simulink model "lab4_3_"  (R2023a)
settings: Solver=VariableStepAuto  StartTime=0.0  StopTime=50  RelTol=1e-3
values from neighbouring files (symbols this model uses):
  kd = 0.48315    [lab4_3.m]
  ki = 1.8463    [lab4_3.m]
  kp = 1.1776    [lab4_3.m]
libraries: checkpacklib x2, slpidlib x1
settings Model: Creator=diontep  LastModifiedBy=diontep

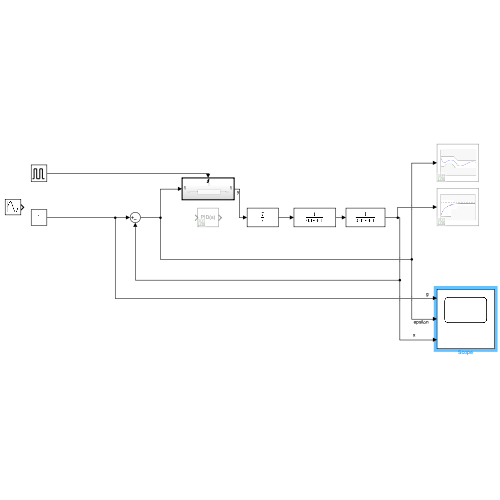
[thumbnail: Simulink's stored preview of the top-level diagram]
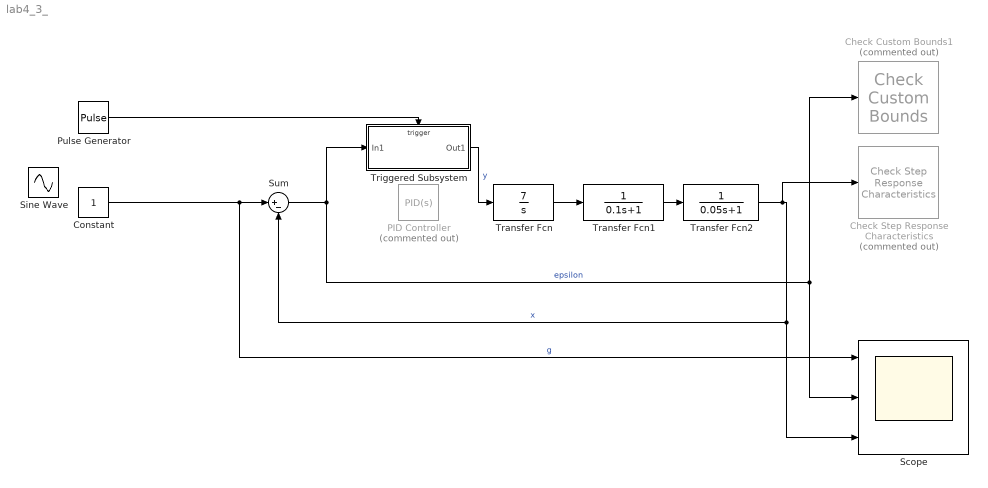
== system lab4_3_ ==
  Check Custom Bounds1 : checkpacklib/Check Custom Bounds  Commented=on  InstantiateOnLoad=on  enabled=on  stopWhenAssertionFail=off  export=off  ViewDlgPos=[]  OpenViewOnLoad=off  LaunchViewOnOpen=off  TimeUnits=seconds  EnableUpperBound=on  UpperBoundTimes=[0 5; 5 50]  UpperBoundAmplitudes=[10 10; 1 1];  EnableLowerBound=on  LowerBoundTimes=[0 5; 5 50]  LowerBoundAmplitudes=[-10 -10; -1 -1];
      settings: LibrarySourceBlock=sdolib/Signal Constraints/Check Custom Bounds
  Check Step Response Characteristics : checkpacklib/Check Step Response  Characteristics  Commented=on  InstantiateOnLoad=on  enabled=on  stopWhenAssertionFail=off  export=off  ViewDlgPos=[]  OpenViewOnLoad=off  LaunchViewOnOpen=off  TimeUnits=seconds  EnableStepResponseBound=on  InitialValue=0  FinalValue=1  StepTime=0  RiseTime=5  PercentRise=80  SettlingTime=7  PercentSettling=1  PercentOvershoot=10  PercentUndershoot=1
      settings: LibrarySourceBlock=|
      | sdolib/Signal Constraints/Check Step Response
      | Characteristics
  Constant : Constant
  PID Controller : slpidlib/PID Controller  Commented=on  Controller=PID  Form=Parallel  TimeDomain=Continuous-time  UseExternalTs=off  SampleTime=-1  IntegratorMethod=Forward Euler  FilterMethod=Forward Euler  ControllerParametersSource=internal  P=kp  I=ki  UseKiTs=off  D=kd  N=100  UseFilter=on  TunerSelectOption=Transfer Function Based (PID Tuner App)  InitialConditionSource=internal  InitialConditionForIntegrator=0  InitialConditionForFilter=0  DifferentiatorICPrevScaledInput=0  ExternalReset=none  TrackingMode=off  Kt=1  LimitOutput=off  SatLimitsSource=internal  UpperSaturationLimit=inf  LowerSaturationLimit=-inf  LinearizeAsGain=on  AntiWindupMode=none  Kb=1  LimitIntegrator=off  UpperIntegratorSaturationLimit=inf  LowerIntegratorSaturationLimit=-inf  POutMin=[]  POutMax=[]  IOutMin=[]  IOutMax=[]  DOutMin=[]  DOutMax=[]  NOutMin=[]  NOutMax=[]  SumOutMin=[]  SumOutMax=[]  SaturationOutMin=[]  SaturationOutMax=[]  PParamMin=[]  PParamMax=[]  IParamMin=[]  IParamMax=[]  DParamMin=[]  DParamMax=[]  NParamMin=[]  NParamMax=[]  KbParamMin=[]  KbParamMax=[]  KtParamMin=[]  KtParamMax=[]  KbOutMin=[]  KbOutMax=[]  KtOutMin=[]  KtOutMax=[]  IntegratorOutMin=[]  IntegratorOutMax=[]  FilterOutMin=[]  FilterOutMax=[]  SumI1OutMin=[]  SumI1OutMax=[]  SumI2OutMin=[]  SumI2OutMax=[]  SumI3OutMin=[]  SumI3OutMax=[]  SumI4OutMin=[]  SumI4OutMax=[]  SumDOutMin=[]  SumDOutMax=[]  DifferentiatorOutMin=[]  DifferentiatorOutMax=[]  FilterDiffOutCoefMin=[]  FilterDiffOutCoefMax=[]  ReciprocalOutMin=[]  ReciprocalOutMax=[]  SumDenOutMin=[]  SumDenOutMax=[]  SumNumOutMin=[]  SumNumOutMax=[]  DivideOutMin=[]  DivideOutMax=[]  UdiffTsProdOutMin=[]  UdiffTsProdOutMax=[]  NTsProdOutMin=[]  NTsProdOutMax=[]  UintegralTsProdOutMin=[]  UintegralTsProdOutMax=[]  UngainTsProdOutMin=[]  UngainTsProdOutMax=[]  ClampingZeroOutDataTypeStr=Inherit: Inherit via back propagation  ClampingZeroOutMin=[]  ClampingZeroOutMax=[]  FilterDenConstantOutDataTypeStr=Inherit: Inherit via back propagation  FilterDenConstantOutMin=[]  FilterDenConstantOutMax=[]  PCopyOutDataTypeStr=Inherit: Inherit via back propagation  PCopyOutMin=[]  PCopyOutMax=[]  NCopyOutDataTypeStr=Inherit: Inherit via back propagation  NCopyOutMin=[]  NCopyOutMax=[]  IntegratorContinuousStateAttributes=''  IntegratorStateMustResolveToSignalObject=off  IntegratorRTWStateStorageClass=Auto  FilterContinuousStateAttributes=''  FilterStateMustResolveToSignalObject=off  FilterRTWStateStorageClass=Auto  ParallelPVariant=InternalParameters  IdealPVariant=Disabled  IVariant=InternalParameters  DVariant=InternalParameters  IntegratorVariant=Continuous  SatVariant=Disabled  AWVariant=Passthrough  PCopyVariant=Disabled  TRVariant=Disabled  FdbkBlocksVariant=Forward  IdealPFdbkVariant=Disabled  SatFdbkVariant=Disabled  DerivativeFilterVariant=ContFilter  NVariant=InternalParameters  NCopyVariant=Disabled  FilterICVariant=InternalICsFilter  IntegratorICVariant=InternalICs  ExternalResetVariant=Disabled  TRSumVariant=Passthrough  SumFdbkVariant=Disabled  SumVariant=Sum_PID  TsampFilterVariant=InternalTs  TsampNgainVariant=Passthrough  TsampIntegralVariant=Disabled_SignalSpec  ExternalSaturationOutDataTypeStr=Inherit: Same as second input
  Pulse Generator : DiscretePulseGenerator  PulseType=Time based  Period=0.01  PulseWidth=50
  Scope : Scope  NumInputPorts=3
  Sine Wave : Sin  Amplitude=50  Frequency=0.5  SampleTime=0
  Sum : Sum  Inputs=|+-
  Transfer Fcn : TransferFcn  Numerator=[7]  Denominator=[1 0]
  Transfer Fcn1 : TransferFcn  Denominator=[0.1 1]
  Transfer Fcn2 : TransferFcn  Denominator=[0.05 1]
  Triggered Subsystem : Subsystem  TreatAsAtomicUnit=on
  wires:
  Sum/1 -> Triggered Subsystem/1(In1), Check Custom Bounds1/1, Scope/2  "epsilon"
  Transfer Fcn/1 -> Transfer Fcn1/1
  Transfer Fcn1/1 -> Transfer Fcn2/1
  Transfer Fcn2/1 -> Check Step Response Characteristics/1, Sum/2, Scope/3  "x"
  Pulse Generator/1 -> Triggered Subsystem/Trigger
  Constant/1 -> Scope/1, Sum/1  "g"
  Triggered Subsystem/1(Out1) -> Transfer Fcn/1  "y"

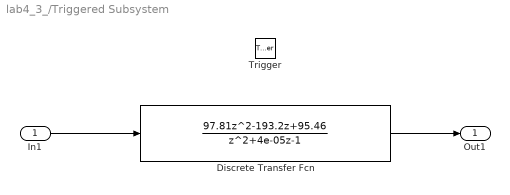
== system lab4_3_/Triggered Subsystem ==
  In1 : Inport
  Trigger : TriggerPort  VariantControl=(inherit)
  Discrete Transfer Fcn : DiscreteTransferFcn  Numerator=[97.81 -193.2 95.46]  Denominator=[1 4e-05 -1]
  Out1 : Outport
  wires:
  In1/1 -> Discrete Transfer Fcn/1
  Discrete Transfer Fcn/1 -> Out1/1
